simulink model "intep"  (R2017b)
settings: Solver=VariableStepAuto  StartTime=0.0  StopTime=5.0  RelTol=1e-3
libraries: simulink x2
settings Model: Creator=kouakam  LastModifiedBy=kouakam

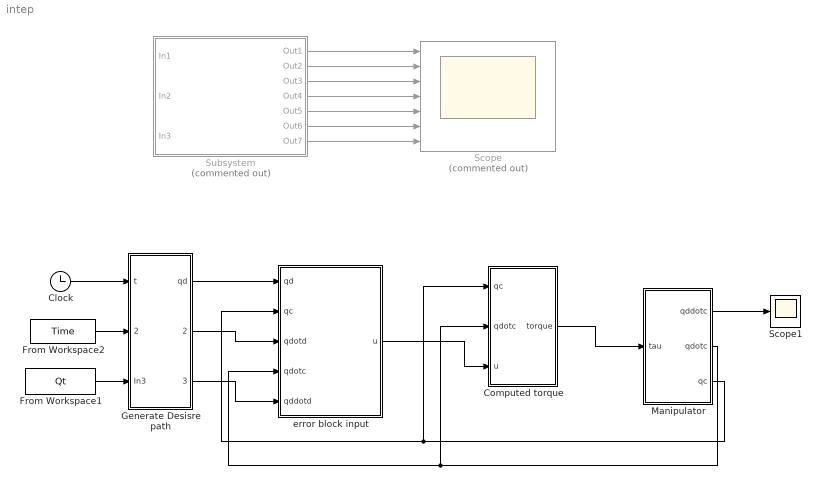
== system intep ==
  Clock : Clock
  Computed torque : Subsystem
  From Workspace1 : FromWorkspace  VariableName=Qt  SampleTime=0
  From Workspace2 : FromWorkspace  VariableName=Time  SampleTime=0
  Generate Desisre path : Subsystem
  Manipulator : Subsystem
  Scope : Scope  Commented=on  NumInputPorts=7
  Scope1 : Scope
  Subsystem : Subsystem  Commented=on
  error block input : Subsystem
  wires:
  Clock/1 -> Generate Desisre path/1("t ")
  From Workspace2/1 -> Generate Desisre path/2(stpan)
  From Workspace1/1 -> Generate Desisre path/3(In3)
  Generate Desisre path/1("qd ") -> error block input/1("qd ")
  Generate Desisre path/2("qdotd ") -> error block input/3("qdotd ")
  Generate Desisre path/3(qddotd) -> error block input/5("qddotd ")
  Manipulator/3(qc) -> Computed torque/1("qc "), error block input/2("qc ")
  Manipulator/2(qdotc) -> Computed torque/2(qdotc), error block input/4(qdotc)
  error block input/1("u ") -> Computed torque/3(u)
  Computed torque/1(torque) -> Manipulator/1(tau)
  Subsystem/6(Out6) -> Scope/6
  Subsystem/7(Out7) -> Scope/7
  Subsystem/2(Out2) -> Scope/2
  Subsystem/5(Out5) -> Scope/5
  Subsystem/1(Out1) -> Scope/1
  Subsystem/3(Out3) -> Scope/3
  Subsystem/4(Out4) -> Scope/4
  Manipulator/1(qddotc) -> Scope1/1

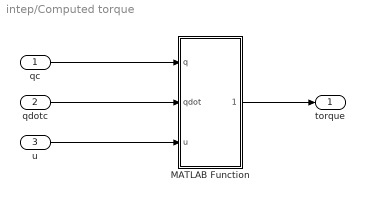
== system intep/Computed torque ==
  "qc " : Inport
  qdotc : Inport  Port=2
  u : Inport  Port=3
  MATLAB Function : MATLAB Function  TreatAsAtomicUnit=on
  torque : Outport
  wires:
  MATLAB Function/1(torque) -> torque/1
  u/1 -> MATLAB Function/3(u)
  "qc "/1 -> MATLAB Function/1(q)
  qdotc/1 -> MATLAB Function/2(qdot)

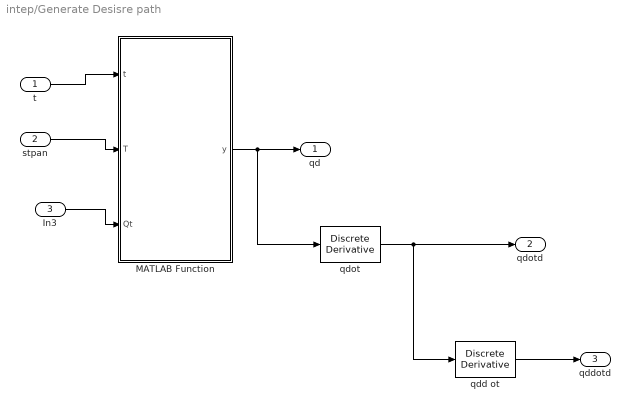
== system intep/Generate Desisre path ==
  "t " : Inport
  stpan : Inport  Port=2
  In3 : Inport  Port=3
  MATLAB Function : MATLAB Function  TreatAsAtomicUnit=on
  qdd ot : simulink/Discrete/Discrete Derivative  gainval=1.0  ICPrevScaledInput=0.0  OutMin=[]  OutMax=[]  OutDataType=fixdt(1, 16)  OutScaling=2^-10  DoSatur=off
  qdot : simulink/Discrete/Discrete Derivative  gainval=1.0  ICPrevScaledInput=0.0  OutMin=[]  OutMax=[]  OutDataType=fixdt(1, 16)  OutScaling=2^-10  DoSatur=off
  "qd " : Outport
  "qdotd " : Outport  Port=2
  qddotd : Outport  Port=3
  wires:
  stpan/1 -> MATLAB Function/2(T)
  In3/1 -> MATLAB Function/3(Qt)
  "t "/1 -> MATLAB Function/1(t)
  MATLAB Function/1(y) -> qdot/1, "qd "/1
  qdot/1 -> qdd ot/1, "qdotd "/1
  qdd ot/1 -> qddotd/1

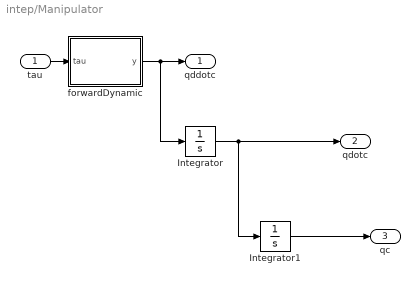
== system intep/Manipulator ==
  tau : Inport
  Integrator : Integrator
  Integrator1 : Integrator
  "forwardDynamic " : MATLAB Function  TreatAsAtomicUnit=on
  qddotc : Outport
  qdotc : Outport  Port=2
  qc : Outport  Port=3
  wires:
  tau/1 -> "forwardDynamic "/1(tau)
  Integrator/1 -> Integrator1/1, qdotc/1
  "forwardDynamic "/1(y) -> Integrator/1, qddotc/1
  Integrator1/1 -> qc/1

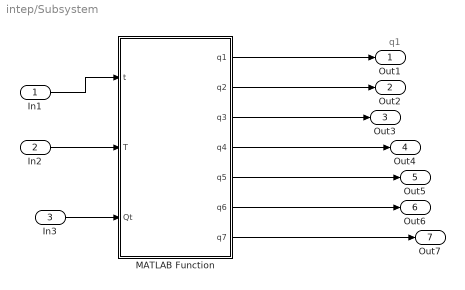
== system intep/Subsystem ==
  note: q1
  In1 : Inport
  In2 : Inport  Port=2
  In3 : Inport  Port=3
  MATLAB Function : MATLAB Function  TreatAsAtomicUnit=on
  Out1 : Outport
  Out2 : Outport  Port=2
  Out3 : Outport  Port=3
  Out4 : Outport  Port=4
  Out5 : Outport  Port=5
  Out6 : Outport  Port=6
  Out7 : Outport  Port=7
  wires:
  MATLAB Function/1(q1) -> Out1/1
  In1/1 -> MATLAB Function/1(t)
  In2/1 -> MATLAB Function/2(T)
  In3/1 -> MATLAB Function/3(Qt)
  MATLAB Function/7(q7) -> Out7/1
  MATLAB Function/6(q6) -> Out6/1
  MATLAB Function/5(q5) -> Out5/1
  MATLAB Function/4(q4) -> Out4/1
  MATLAB Function/3(q3) -> Out3/1
  MATLAB Function/2(q2) -> Out2/1

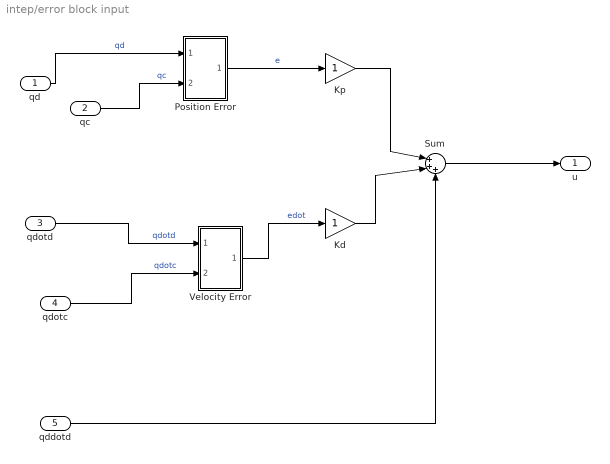
== system intep/error block input ==
  "qd " : Inport
  "qc " : Inport  Port=2
  "qdotd " : Inport  Port=3
  qdotc : Inport  Port=4
  "qddotd " : Inport  Port=5
  "Kd " : Gain
  "Kp " : Gain
  Position Error : Subsystem
  Sum : Sum  Inputs=|+++
  Velocity Error : Subsystem
  "u " : Outport
  wires:
  "qc "/1 -> Position Error/2(In2)  "qc"
  qdotc/1 -> Velocity Error/2(In2)  "qdotc"
  "qd "/1 -> Position Error/1(In1)  "qd"
  "qdotd "/1 -> Velocity Error/1(In1)  "qdotd"
  Position Error/1(Out1) -> "Kp "/1  "e"
  Velocity Error/1(Out1) -> "Kd "/1  "edot"
  "qddotd "/1 -> Sum/3
  Sum/1 -> "u "/1
  "Kp "/1 -> Sum/1
  "Kd "/1 -> Sum/2

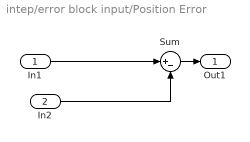
== system intep/error block input/Position Error ==
  In1 : Inport
  In2 : Inport  Port=2
  Sum : Sum  Inputs=|+-
  Out1 : Outport
  wires:
  In2/1 -> Sum/2
  Sum/1 -> Out1/1
  In1/1 -> Sum/1

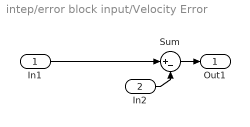
== system intep/error block input/Velocity Error ==
  In1 : Inport
  In2 : Inport  Port=2
  Sum : Sum  Inputs=|+-
  Out1 : Outport
  wires:
  In2/1 -> Sum/2
  Sum/1 -> Out1/1
  In1/1 -> Sum/1

== matlab function intep/Generate Desisre path/MATLAB Function ==
  data: t input; y output; T input; Qt input
function y  =  fcn(  t, T, Qt)

q1 = interp1(T,Qt(1,:),t,'nearest');
q2 = interp1(T,Qt(2,:),t,'nearest');
q3 = interp1(T,Qt(3,:),t,'nearest');
q4 = interp1(T,Qt(4,:),t,'nearest');
q5 = interp1(T,Qt(5,:),t,'nearest');
q6 = interp1(T,Qt(6,:),t,'nearest');
q7 = interp1(T,Qt(7,:),t,'nearest');
y=[q1,q2,q3,q4,q5,q6,q7];

== matlab function intep/Subsystem/MATLAB Function ==
  data: t input; q1 output; q2 output; q3 output; q4 output; q5 output; q6 output; T input; Qt input; q7 output
function [q1,q2,q3, q4,q5,q6,q7] =  fcn(  t, T, Qt)

q1 = interp1(T,Qt(1,:),t,'nearest');
q2 = interp1(T,Qt(2,:),t,'nearest');
q3 = interp1(T,Qt(3,:),t,'nearest');
q4 = interp1(T,Qt(4,:),t,'nearest');
q5 = interp1(T,Qt(5,:),t,'nearest');
q6 = interp1(T,Qt(6,:),t,'nearest');
q7 = interp1(T,Qt(7,:),t,'nearest');

== matlab function intep/Computed torque/MATLAB Function ==
  data: q input size=[1 7]; qdot input size=[1 7]; u input size=[1 7]; torque output double size=[1 7]
function torque = fcn(q, qdot, u)

lbr  = exampleHelperMwIiwa14();
tau =lbr.inverseDynamics(q,qdot,u);
torque = tau;

== matlab function intep/Manipulator/forwardDynamic  ==
  data: tau input; y output size=[1 7]
function y = fcn(tau)

 lbr = exampleHelperMwIiwa14();

  qddot=lbr.forwardDynamics([],[],tau');
y = qddot;
